simulink model "six"  (R2020b)
settings: Solver=VariableStepAuto  StartTime=0.0  StopTime=10.0  RelTol=1e-3
settings Model: Creator=Dell  LastModifiedBy=Dell

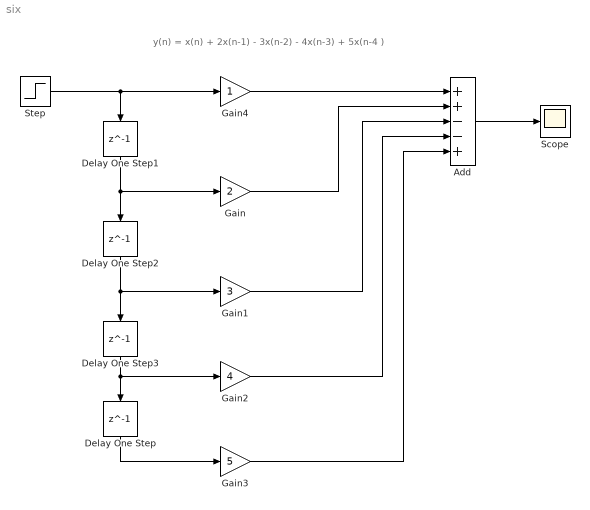
== system six ==
  note: y(n) = x(n) + 2x(n-1) - 3x(n-2) - 4x(n-3) + 5x(n-4 )
  Add : Sum  Inputs=++--+
  Delay One Step{,1..3} (4 alike) : Delay  DelayLength=1
  Gain : Gain  Gain=2
  Gain1 : Gain  Gain=3
  Gain2 : Gain  Gain=4
  Gain3 : Gain  Gain=5
  Gain4 : Gain
  Scope : Scope
  Step : Step  SampleTime=0
  wires:
  Step/1 -> Delay One Step1/1, Gain4/1
  Delay One Step1/1 -> Gain/1, Delay One Step2/1
  Delay One Step2/1 -> Gain1/1, Delay One Step3/1
  Delay One Step3/1 -> Delay One Step/1, Gain2/1
  Delay One Step/1 -> Gain3/1
  Gain4/1 -> Add/1
  Gain/1 -> Add/2
  Gain1/1 -> Add/3
  Gain2/1 -> Add/4
  Gain3/1 -> Add/5
  Add/1 -> Scope/1
